simulink subsystem "SelfDefined_Boost_Converter"  (R2024b)
settings: Solver=VariableStepAuto  StartTime=0.0  StopTime=10.0  RelTol=1e-3
libraries: simulink x1, spsDiodeLib x1, spsIGBTLib x1
settings Model: Creator=XixiLab  LastModifiedBy=XixiLab

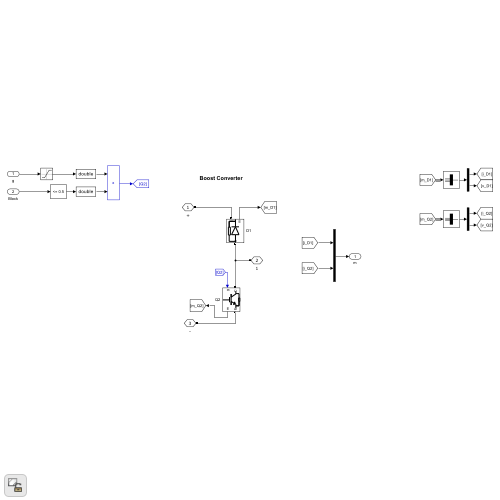
[thumbnail: Simulink's stored preview of the top-level diagram]
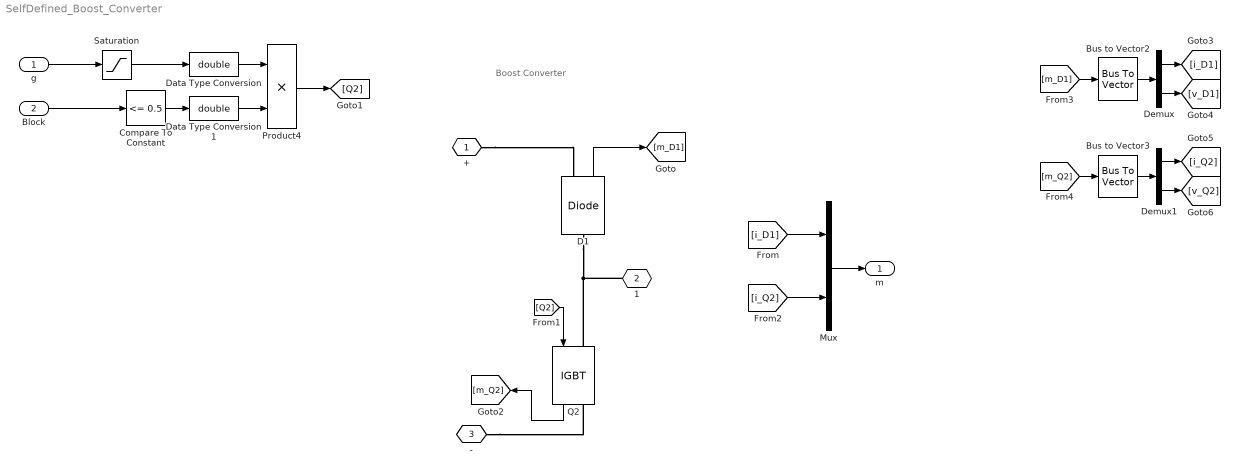
== system SelfDefined_Boost_Converter ==
  note: Boost Converter
  g : Inport  PortDimensions=1
  Block : Inport  Port=2  PortDimensions=1
  Bus to Vector2 : BusToVector
  Bus to Vector3 : BusToVector
  Compare To Constant : simulink/Logic and Bit Operations/Compare To Constant  relop=<=  const=0.5  OutDataTypeStr=boolean
  D1 : spsDiodeLib/Diode  Ron=0.001  Lon=0  Vf=0  IC=0  UseSnubber=0  Rs=1e6  Cs=inf  Measurements=on
  Data Type Conversion : DataTypeConversion  OutDataTypeStr=double  SaturateOnIntegerOverflow=off  RndMeth=Floor
  Data Type Conversion1 : DataTypeConversion  OutDataTypeStr=double  SaturateOnIntegerOverflow=off  RndMeth=Floor
  Demux : Demux  Outputs=2
  Demux1 : Demux  Outputs=2
  Mux : Mux  Inputs=2
  Product4 : Product
  Q2 : spsIGBTLib/IGBT  Ron=0.001  Lon=0  Vf=0  Tf=1e-6  Tt=2e-6  IC=0  Rs=1e6  Cs=inf  Measurements=on
  Saturation : Saturate  UpperLimit=1  LowerLimit=0
  + : PMIOPort  Tag=PMCPort  Side=Right
  1 : PMIOPort  Tag=PMCPort  Port=2  Side=Left
  - : PMIOPort  Tag=PMCPort  Port=3  Side=Right
  m : Outport
  wires:
  [Q2] -> Q2/1
  Data Type Conversion/1 -> Product4/1
  Block/1 -> Compare To Constant/1
  Saturation/1 -> Data Type Conversion/1
  Data Type Conversion1/1 -> Product4/2
  Product4/1 -> [Q2]
  Compare To Constant/1 -> Data Type Conversion1/1
  g/1 -> Saturation/1
  D1/1 -> [m_D1]
  Q2/1 -> [m_Q2]
  Mux/1 -> m/1
  [i_D1] -> Mux/1
  [i_Q2] -> Mux/2
  [m_D1] -> Bus to Vector2/1
  [m_Q2] -> Bus to Vector3/1
  Bus to Vector2/1 -> Demux/1
  Demux/1 -> [i_D1]
  Demux/2 -> [v_D1]
  Bus to Vector3/1 -> Demux1/1
  Demux1/1 -> [i_Q2]
  Demux1/2 -> [v_Q2]
  connections:
  1/RConn1 -- Q2/LConn1 -- D1/LConn1
  -/RConn1 -- Q2/RConn1
  +/RConn1 -- D1/RConn1
